simulink model "bicopter_fuzzy"  (R2022b)
settings: Solver=VariableStepAuto  StartTime=0.0  StopTime=20.0  RelTol=1e-3
libraries: fuzblock x2
settings Model: Creator=KIIT  LastModifiedBy=KIIT
settings DebuggingCC: UnconnectedInputMsg=warning  UnconnectedOutputMsg=warning  UnconnectedLineMsg=warning
settings ModelReferenceCC: EnableRefExpFcnMdlSchedulingChecks=on
settings RTWCC: DLArmComputeVersion=19.05

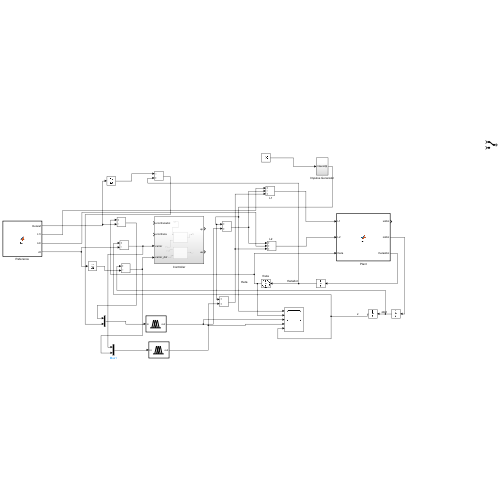
[thumbnail: Simulink's stored preview of the top-level diagram]
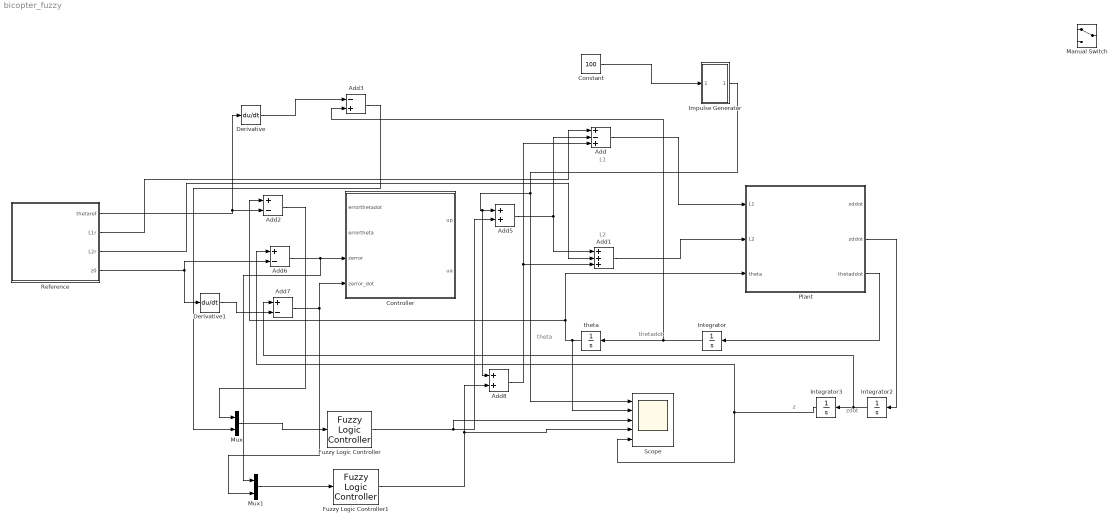
== system bicopter_fuzzy ==
  note: z
  note: zdot
  note: L2
  note: L1
  note: theta
  note: thetadot
  Add : Sum  Inputs=+-+
  Add1 : Sum  Inputs=+++
  Add2 : Sum  Inputs=+-
  Add3 : Sum  Inputs=-+
  Add5 : Sum
  Add6 : Sum  Inputs=+-
  Add7 : Sum  Inputs=+-
  Add8 : Sum
  Constant : Constant  Value=100
  Controller : Subsystem
  Derivative : Derivative
  Derivative1 : Derivative
  Fuzzy Logic Controller : fuzblock/Fuzzy Logic  Controller  FIS=cpFIS  OutputSampleNumber=101  DataType=double  FuzzifiedInputs=off  RuleFiringStrengths=off  RuleOutputs=off  AggregatedOutputs=off  SimulateUsing=Interpreted execution  OutOfRangeInputValueMessage=warning  NoRuleFiredMessage=warning  EmptyOutputFuzzySetMessage=warning
  Fuzzy Logic Controller1 : fuzblock/Fuzzy Logic  Controller  FIS=cplFIS  OutputSampleNumber=101  DataType=double  FuzzifiedInputs=off  RuleFiringStrengths=off  RuleOutputs=off  AggregatedOutputs=off  SimulateUsing=Interpreted execution  OutOfRangeInputValueMessage=warning  NoRuleFiredMessage=warning  EmptyOutputFuzzySetMessage=warning
  Impulse Generator : Subsystem
  Integrator : Integrator
  Integrator2 : Integrator
  Integrator3 : Integrator
  Manual Switch : ManualSwitch
  Mux : Mux  Inputs=2
  Mux1 : Mux  Inputs=2
  Plant : MATLAB Function  TreatAsAtomicUnit=on
  Reference : MATLAB Function  TreatAsAtomicUnit=on
  Scope : Scope  NumInputPorts=5
  theta : Integrator  InitialCondition=pi/6.0  WrapState=on
  wires:
  Reference/2(L1r) -> Add/1
  Reference/3(L2r) -> Add1/2
  Add/1 -> Plant/1(L1)
  Add1/1 -> Plant/2(L2)
  Plant/3(thetaddot) -> Integrator/1
  Integrator/1 -> Add3/2, theta/1
  theta/1 -> Scope/2, Plant/3(theta), Add2/1
  Reference/1(thetaref) -> Add2/2, Derivative/1
  Derivative/1 -> Add3/1
  Add5/1 -> Add/2, Add1/1
  Plant/2(zddot) -> Integrator2/1
  Integrator2/1 -> Add7/1, Integrator3/1
  Reference/4(z0) -> Derivative1/1, Add6/2
  Integrator3/1 -> Scope/5, Add6/1
  Derivative1/1 -> Add7/2
  Add8/1 -> Add/3, Add1/3
  Impulse Generator/1(Out1) -> Scope/1, Add8/1, Add5/1
  Add6/1 -> Mux1/1, Controller/3(zerror)
  Add7/1 -> Controller/4(zerror_dot), Mux1/2
  Fuzzy Logic Controller/1 -> Scope/3, Add5/2
  Mux/1 -> Fuzzy Logic Controller/1
  Constant/1 -> Impulse Generator/1(Intensity)
  Mux1/1 -> Fuzzy Logic Controller1/1
  Add3/1 -> Mux/2
  Add2/1 -> Mux/1
  Fuzzy Logic Controller1/1 -> Scope/4, Add8/2

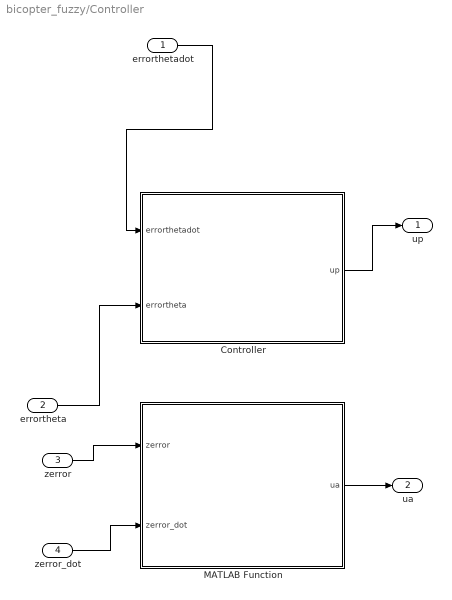
== system bicopter_fuzzy/Controller ==
  errorthetadot : Inport
  errortheta : Inport  Port=2
  zerror : Inport  Port=3
  zerror_dot : Inport  Port=4
  Controller : MATLAB Function  TreatAsAtomicUnit=on
  MATLAB Function : MATLAB Function  TreatAsAtomicUnit=on
  up : Outport
  ua : Outport  Port=2
  wires:
  errortheta/1 -> Controller/2(errortheta)
  MATLAB Function/1(ua) -> ua/1
  errorthetadot/1 -> Controller/1(errorthetadot)
  zerror/1 -> MATLAB Function/1(zerror)
  Controller/1(up) -> up/1
  zerror_dot/1 -> MATLAB Function/2(zerror_dot)

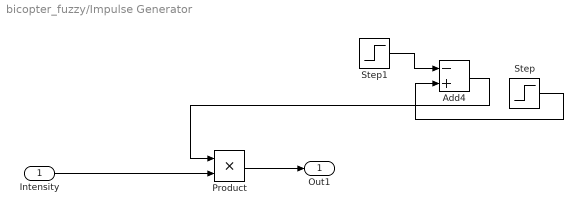
== system bicopter_fuzzy/Impulse Generator ==
  Intensity : Inport
  Add4 : Sum  Inputs=-+
  Product : Product
  Step : Step  SampleTime=0
  Step1 : Step  Time=2  SampleTime=0
  Out1 : Outport
  wires:
  Step1/1 -> Add4/1
  Step/1 -> Add4/2
  Add4/1 -> Product/1
  Product/1 -> Out1/1
  Intensity/1 -> Product/2

== matlab function bicopter_fuzzy/Plant ==
  data: L1 input; xddot output; L2 input; theta input; zddot output; thetaddot output
function [xddot, zddot, thetaddot] = fcn(L1, L2, theta)
m = 2;
Iy = 0.2;
g = 9.8;
d = 0.2;
k1 = 24;
k2 = 7;
o1 = -(1/m)*(L1+L2)*sin(theta);
o2 = (1/m)*(m*g - (L1+L2)*cos(theta));
o3 =(1/Iy)*d*(L1-L2);
xddot = o1;
zddot = o2;
thetaddot = o3;

== matlab function bicopter_fuzzy/Controller/Controller ==
  data: errorthetadot input; up output; errortheta input
function up  = fcn(errorthetadot, errortheta)
m = 2;
Iy = 0.2;
g = 9.8;
d = 0.2;
k1 = 24;
k2 = 7;
up = (Iy/(2*d))*((1+k1)*errortheta + k2*errorthetadot);

== matlab function bicopter_fuzzy/Reference ==
  data: thetaref output; L1r output; L2r output; z0 output
function [thetaref, L1r, L2r, z0] = fcn()
m = 2;
Iy = 0.2;
g = 9.8;
d = 0.2;
k1 = 24;
k2 = 7;
u = [0, m*g/2, m*g/2];
thetaref = 0;
L1r = m*g/2;
L2r = m*g/2;
z0 = 40;

== matlab function bicopter_fuzzy/Controller/MATLAB Function ==
  data: zerror input; ua output; zerror_dot input
function ua = fcn(zerror,zerror_dot)
m = 2;
g = 9.8;
d = 0.2;
k3 = 3;
k4 = 3;
ubar = m*((1+k3)*zerror+k4*zerror_dot);
ua = ubar/2.0;
